simulink model "tuning"  (R2024b)
settings: Solver=FixedStepAuto  StartTime=0.0  StopTime=3  FixedStep=1e-6  RelTol=1e-3
values from neighbouring files (symbols this model uses):
  BW_out = BW_out_DC    [main.m]
  C_filt = parameter.Value(6)    [main.m]
  closedL_P = feedback(openL_P, 1)    [main.m]
  closedL_V = feedback(openL_V, 1)    [main.m]
  DC = 1    [main.m]
  I_charge = C_dc * Vdc_base / t_charge    [main.m]
  inner_loop = collect(-I_V1/V1, "s")    [scam.m]
  ki_outer = ki_outer_DC_pu    [main.m]
  kp_outer = kp_outer_DC_pu    [main.m]
  L_base = Z_base / omega_b    [main.m]
  L_vsc = parameter.Value(5)    [main.m]
  omega_b = 2 * pi * f_base    [main.m]
  P_base = parameter.Value(4)*10^6    [main.m]
  Pm_out = Pm_out_DC    [main.m]
  Power = 0    [main.m]
  R_filt = parameter.Value(8)    [main.m]
  R_vsc = parameter.Value(7)    [main.m]
  t_charge = 0.5    [main.m]
  Ts = parameter.Value(1)*10^-6    [main.m]
  V_base = parameter.Value(3)*10^3    [main.m]
undefined symbols (not defined in the file or in its folder): BW_in, BW_out_DC, BW_out_P, BW_out_V, BW_pll, C_dc, ki_inner_pu, ki_outer_DC_pu, ki_outer_P_pu, ki_outer_V_pu, ki_pll, kp_inner_pu, kp_outer_DC_pu, kp_outer_P_pu, kp_outer_V_pu, kp_pll, L, L_grid, openL_DC, Pm_out_DC, Pm_out_P, Pm_out_V, Pm_pll, R_grid, tau_max, Vdc_base
libraries: slpidlib x5, spsabctodq0Lib x4, spsControlledVoltageSourceLib x3, spsControlledCurrentSourceLib x2, eeGeneralControl x2, spsThreePhaseSeriesRLCBranchLib x2, spsThreePhaseVIMeasurementLib x2, spsGroundLib x1, spsParallelRLCBranchLib x1, spsThreePhaseSourceLib x1, spsVoltageMeasurementLib x1, spsdq0toabcLib x1
settings Model: Creator=osro  LastModifiedBy=nicolae.darii
settings SolverCC: AlgebraicLoopSolver=TrustRegion
settings DebuggingCC: UnconnectedInputMsg=warning  UnconnectedOutputMsg=warning  UnconnectedLineMsg=warning
settings ModelReferenceCC: EnableRefExpFcnMdlSchedulingChecks=on
settings RTWCC: GPUComputeCapability=3.5

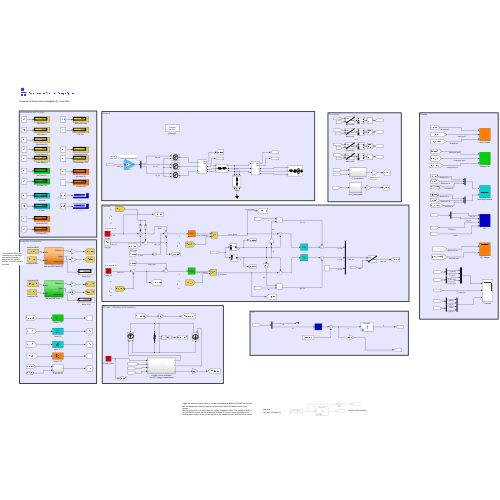
[thumbnail: Simulink's stored preview of the top-level diagram]
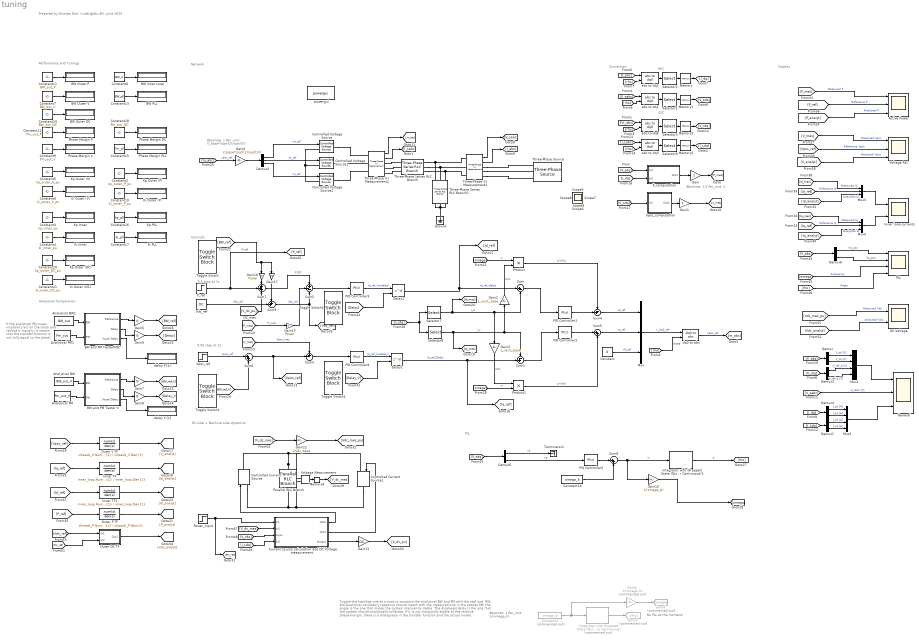
== system tuning ==
  note: PLL
  note: Toggle the switches one at a time to compare the analytical BW and PM with the real one:
      | BW: the analytical oscillatory responce should match with the measured one in the scopes
      | PM: the angle is the one that makes the system margianlly stable. The displayed delay is the one that the system should analytically tollerate. If it is not margianlly stable at the relative phase-margin, there is a divergnece in the transfer function and the actual model.
  note: If the analytical PM cuses instability act on the block and reduce it maualy (it means that the transfer function is not fully equal to the plant)
  note: No PLL at the moment!
  note: 0.05 step at 2s
  note: 0.5 step at 1s
  note: Absolute: 1
      | Per_unit: 1/(omega_b)
  note: Absolute: 1.5
      | Per_unit: 1
  note: Absolute: 1
      | Per_unit: V_base*(sqrt(2)/sqrt(3))
  note: Display
  note: Conversion
  note: Controls
  note: Analytical Comparision
  note: Network
  note: Performance and Tunings
  note: VSC
  note: PoC
  note: Prepared by Nicolae Darii (nidar@dtu.dk), June 2025
  note: DC side + Machine side dynamics
  Active Power : Scope  NumInputPorts=3
  Analytical BW : Constant  Value=BW_out_V
  Analytical BW1 : Constant  Value=BW_out
  Analytical PM : Constant  Value=Pm_out_V
  Analytical PM1 : Constant  Value=Pm_out
  BW Inner Loop : Display
  BW Outer DC : Display
  BW Outer P : Display
  BW Outer V : Display
  BW PLL : Display
  BW and PM Tester V : Subsystem
  BW and PM TesterP/DC : Subsystem
  Constant : Constant  Value=0
  Constant1 : Constant  Commented=on  Value=omega_b
  Constant10 : Constant  Value=ki_outer_P_pu
  Constant11 : Constant  Value=BW_out_P
  Constant12 : Constant  Value=Pm_out_P
  Constant13 : Constant  Value=BW_pll
  Constant14 : Constant  Value=omega_b
  Constant15 : Constant  Value=Pm_pll
  Constant16 : Constant  Value=kp_pll
  Constant17 : Constant  Value=ki_pll
  Constant18 : Constant  Value=Pm_out_DC
  Constant19 : Constant  Value=BW_out_DC
  Constant2 : Constant  Value=kp_outer_P_pu
  Constant20 : Constant  Value=kp_outer_DC_pu
  Constant21 : Constant  Value=ki_outer_DC_pu
  Constant3 : Constant  Value=kp_inner_pu
  Constant4 : Constant  Value=ki_inner_pu
  Constant5 : Constant  Value=kp_outer_V_pu
  Constant6 : Constant  Value=ki_outer_V_pu
  Constant7 : Constant  Value=BW_out_V
  Constant8 : Constant  Value=BW_in
  Constant9 : Constant  Value=Pm_out_V
  Controlled Current Source : spsControlledCurrentSourceLib/Controlled Current Source  Initialize=on  Source_Type=AC  Amplitude=0  Phase=0  Frequency=0  Measurements=None
  Controlled Current Source1 : spsControlledCurrentSourceLib/Controlled Current Source  Initialize=on  Source_Type=AC  Amplitude=0  Phase=0  Frequency=0  Measurements=None
  Controlled Voltage Source : spsControlledVoltageSourceLib/Controlled Voltage Source  Initialize=on  Source_Type=AC  Amplitude=0  Phase=0  Frequency=0  Measurements=None
  Controlled Voltage Source1 : spsControlledVoltageSourceLib/Controlled Voltage Source  Initialize=on  Source_Type=AC  Amplitude=0  Phase=0  Frequency=0  Measurements=None
  Controlled Voltage Source2 : spsControlledVoltageSourceLib/Controlled Voltage Source  Initialize=on  Source_Type=AC  Amplitude=0  Phase=0  Frequency=0  Measurements=None
  Current source calculation and DC Voltage measurement : Subsystem
  DC Voltage : Scope  NumInputPorts=2
  Delay1 : Delay  DelayLengthSource=Input port  DelayLength=floor(tau_max/Ts)  DelayLengthUpperLimit=10000
      settings: InputPortMap=u0,p1
  Delay2 : Delay  DelayLengthSource=Input port  DelayLength=floor(tau_max/Ts)  DelayLengthUpperLimit=10000
      settings: InputPortMap=u0,p1
  Demux{,1,3..6} (6 alike) : Demux  Outputs=2
  Demux2 : Demux  Outputs=3
  Gain : Gain
  Gain1 : Gain
  Gain10 : Gain  Gain=1/(omega_b)
  Gain11 : Gain  Gain=DC
  Gain12 : Gain  Gain=1/Vdc_base
  Gain13 : Gain  Gain=Power
  Gain16 : Gain  Gain=Power
  Gain17 : Gain  Gain=DC
  Gain2 : Gain  Gain=L_vsc/L_base
  Gain3 : Gain  Gain=L_vsc/L_base
  Gain4 : Gain  Commented=on  Gain=1/(omega_b)
  Gain{5,7..9} (4 alike) : Gain  Gain=0
  Gain6 : Gain  Gain=V_base*(sqrt(2)/sqrt(3))
  General : Scope  NumInputPorts=3
  Goto3 : Goto  Commented=on  GotoTag=rho
  Goto4 : Goto  Commented=on  GotoTag=omega
  Ground : spsGroundLib/Ground  LConnTagsString=a
  Inner TF : TransferFcn  Numerator=inner_loop.Num{1}  Denominator=inner_loop.Den{1}
  Inner TF1 : TransferFcn  Numerator=inner_loop.Num{1}  Denominator=inner_loop.Den{1}
  Inner loop currents : Scope  NumInputPorts=2
  Integrator with Wrapped State (Discrete or Continuous) : eeGeneralControl/Integrator with Wrapped State (Discrete or Continuous)  Commented=on  LabelModeActiveChoice=Discrete  WrappedStateUpperValue=2*pi  WrappedStateLowerValue=0  x0=0  Ts=-1
  Integrator with Wrapped State (Discrete or Continuous)1 : eeGeneralControl/Integrator with Wrapped State (Discrete or Continuous)  LabelModeActiveChoice=Discrete  WrappedStateUpperValue=2*pi  WrappedStateLowerValue=0  x0=0  Ts=-1
  Ki Inner : Display
  Ki Outer (DC) : Display
  Ki Outer (P) : Display
  Ki Outer (V) : Display
  Ki PLL : Display
  Kp Inner : Display
  Kp Outer (DC) : Display
  Kp Outer (P) : Display
  Kp Outer (V) : Display
  Kp PLL : Display
  Memory{,1..3} (4 alike) : Memory  InitialCondition=[0 0]  InheritSampleTime=on  LinearizeMemory=on  LinearizeAsDelay=on
  Memory4 : Memory
  Mux : Mux  Inputs=3
  Mux1 : Mux
  Mux2 : Mux
  Mux3 : Mux  Inputs=3
  Mux4 : Mux  Inputs=3
  Outer DC TF : Subsystem
  Outer P TF : TransferFcn  Numerator=closedL_P.Num{1}  Denominator=closedL_P.Den{1}
  Outer V TF : TransferFcn  Numerator=closedL_V.Num{1}  Denominator=closedL_V.Den{1}
  PID Controller1 : slpidlib/PID Controller  Controller=PI  Form=Parallel  TimeDomain=Discrete-time  UseExternalTs=off  SampleTime=Ts  IntegratorMethod=Forward Euler  FilterMethod=Forward Euler  ControllerParametersSource=internal  P=kp_inner_pu  I=ki_inner_pu  UseKiTs=off  D=0  UseExternalDerivativeSource=off  N=100  UseFilter=on  TunerSelectOption=Transfer Function Based (PID Tuner App)  InitialConditionSource=internal  InitialConditionForIntegrator=0  InitialConditionForFilter=0  DifferentiatorICPrevScaledInput=0  ExternalReset=none  TrackingMode=off  Kt=1  LimitOutput=off  SatLimitsSource=internal  UpperSaturationLimit=inf  LowerSaturationLimit=-inf  LinearizeAsGain=on  AntiWindupMode=none  Kb=1  LimitIntegrator=off  UpperIntegratorSaturationLimit=inf  LowerIntegratorSaturationLimit=-inf  POutMin=[]  POutMax=[]  IOutMin=[]  IOutMax=[]  DOutMin=[]  DOutMax=[]  NOutMin=[]  NOutMax=[]  SumOutMin=[]  SumOutMax=[]  SaturationOutMin=[]  SaturationOutMax=[]  PParamMin=[]  PParamMax=[]  IParamMin=[]  IParamMax=[]  DParamMin=[]  DParamMax=[]  NParamMin=[]  NParamMax=[]  KbParamMin=[]  KbParamMax=[]  KtParamMin=[]  KtParamMax=[]  KbOutMin=[]  KbOutMax=[]  KtOutMin=[]  KtOutMax=[]  IntegratorOutMin=[]  IntegratorOutMax=[]  FilterOutMin=[]  FilterOutMax=[]  SumI1OutMin=[]  SumI1OutMax=[]  SumI2OutMin=[]  SumI2OutMax=[]  SumI3OutMin=[]  SumI3OutMax=[]  SumI4OutMin=[]  SumI4OutMax=[]  SumDOutMin=[]  SumDOutMax=[]  DifferentiatorOutMin=[]  DifferentiatorOutMax=[]  FilterDiffOutCoefMin=[]  FilterDiffOutCoefMax=[]  ReciprocalOutMin=[]  ReciprocalOutMax=[]  SumDenOutMin=[]  SumDenOutMax=[]  SumNumOutMin=[]  SumNumOutMax=[]  DivideOutMin=[]  DivideOutMax=[]  UdiffTsProdOutMin=[]  UdiffTsProdOutMax=[]  NTsProdOutMin=[]  NTsProdOutMax=[]  UintegralTsProdOutMin=[]  UintegralTsProdOutMax=[]  UngainTsProdOutMin=[]  UngainTsProdOutMax=[]  ClampingZeroOutDataTypeStr=Inherit: Inherit via back propagation  ClampingZeroOutMin=[]  ClampingZeroOutMax=[]  FilterDenConstantOutDataTypeStr=Inherit: Inherit via back propagation  FilterDenConstantOutMin=[]  FilterDenConstantOutMax=[]  PCopyOutDataTypeStr=Inherit: Inherit via back propagation  PCopyOutMin=[]  PCopyOutMax=[]  NCopyOutDataTypeStr=Inherit: Inherit via back propagation  NCopyOutMin=[]  NCopyOutMax=[]  IntegratorContinuousStateAttributes=''  IntegratorStateMustResolveToSignalObject=off  IntegratorRTWStateStorageClass=Auto  FilterContinuousStateAttributes=''  FilterStateMustResolveToSignalObject=off  FilterRTWStateStorageClass=Auto  ParallelPVariant=InternalParameters  IdealPVariant=Disabled  IVariant=InternalParameters  DVariant=Disabled  IntegratorVariant=Discrete  SatVariant=Disabled  AWVariant=Passthrough  PCopyVariant=Disabled  TRVariant=Disabled  FdbkBlocksVariant=Forward  IdealPFdbkVariant=Disabled  SatFdbkVariant=Disabled  DerivativeFilterVariant=Disabled  NVariant=Disabled  NCopyVariant=Disabled_SignalSpec  FilterICVariant=Disabled  IntegratorICVariant=InternalICs  ExternalResetVariant=Disabled  TRSumVariant=Passthrough  SumFdbkVariant=Disabled  SumVariant=Sum_PI  TsampFilterVariant=InternalTs  TsampNgainVariant=Passthrough  TsampIntegralVariant=Disabled_SignalSpec  ExternalSaturationOutDataTypeStr=Inherit: Same as second input  DerivativeSourceVariant=Disabled  PreIntVariant=InternalPreInt
  PID Controller2 : slpidlib/PID Controller  Controller=PI  Form=Parallel  TimeDomain=Discrete-time  UseExternalTs=off  SampleTime=Ts  IntegratorMethod=Forward Euler  FilterMethod=Forward Euler  ControllerParametersSource=internal  P=kp_inner_pu  I=ki_inner_pu  UseKiTs=off  D=0  UseExternalDerivativeSource=off  N=100  UseFilter=on  TunerSelectOption=Transfer Function Based (PID Tuner App)  InitialConditionSource=internal  InitialConditionForIntegrator=0  InitialConditionForFilter=0  DifferentiatorICPrevScaledInput=0  ExternalReset=none  TrackingMode=off  Kt=1  LimitOutput=off  SatLimitsSource=internal  UpperSaturationLimit=inf  LowerSaturationLimit=-inf  LinearizeAsGain=on  AntiWindupMode=none  Kb=1  LimitIntegrator=off  UpperIntegratorSaturationLimit=inf  LowerIntegratorSaturationLimit=-inf  POutMin=[]  POutMax=[]  IOutMin=[]  IOutMax=[]  DOutMin=[]  DOutMax=[]  NOutMin=[]  NOutMax=[]  SumOutMin=[]  SumOutMax=[]  SaturationOutMin=[]  SaturationOutMax=[]  PParamMin=[]  PParamMax=[]  IParamMin=[]  IParamMax=[]  DParamMin=[]  DParamMax=[]  NParamMin=[]  NParamMax=[]  KbParamMin=[]  KbParamMax=[]  KtParamMin=[]  KtParamMax=[]  KbOutMin=[]  KbOutMax=[]  KtOutMin=[]  KtOutMax=[]  IntegratorOutMin=[]  IntegratorOutMax=[]  FilterOutMin=[]  FilterOutMax=[]  SumI1OutMin=[]  SumI1OutMax=[]  SumI2OutMin=[]  SumI2OutMax=[]  SumI3OutMin=[]  SumI3OutMax=[]  SumI4OutMin=[]  SumI4OutMax=[]  SumDOutMin=[]  SumDOutMax=[]  DifferentiatorOutMin=[]  DifferentiatorOutMax=[]  FilterDiffOutCoefMin=[]  FilterDiffOutCoefMax=[]  ReciprocalOutMin=[]  ReciprocalOutMax=[]  SumDenOutMin=[]  SumDenOutMax=[]  SumNumOutMin=[]  SumNumOutMax=[]  DivideOutMin=[]  DivideOutMax=[]  UdiffTsProdOutMin=[]  UdiffTsProdOutMax=[]  NTsProdOutMin=[]  NTsProdOutMax=[]  UintegralTsProdOutMin=[]  UintegralTsProdOutMax=[]  UngainTsProdOutMin=[]  UngainTsProdOutMax=[]  ClampingZeroOutDataTypeStr=Inherit: Inherit via back propagation  ClampingZeroOutMin=[]  ClampingZeroOutMax=[]  FilterDenConstantOutDataTypeStr=Inherit: Inherit via back propagation  FilterDenConstantOutMin=[]  FilterDenConstantOutMax=[]  PCopyOutDataTypeStr=Inherit: Inherit via back propagation  PCopyOutMin=[]  PCopyOutMax=[]  NCopyOutDataTypeStr=Inherit: Inherit via back propagation  NCopyOutMin=[]  NCopyOutMax=[]  IntegratorContinuousStateAttributes=''  IntegratorStateMustResolveToSignalObject=off  IntegratorRTWStateStorageClass=Auto  FilterContinuousStateAttributes=''  FilterStateMustResolveToSignalObject=off  FilterRTWStateStorageClass=Auto  ParallelPVariant=InternalParameters  IdealPVariant=Disabled  IVariant=InternalParameters  DVariant=Disabled  IntegratorVariant=Discrete  SatVariant=Disabled  AWVariant=Passthrough  PCopyVariant=Disabled  TRVariant=Disabled  FdbkBlocksVariant=Forward  IdealPFdbkVariant=Disabled  SatFdbkVariant=Disabled  DerivativeFilterVariant=Disabled  NVariant=Disabled  NCopyVariant=Disabled_SignalSpec  FilterICVariant=Disabled  IntegratorICVariant=InternalICs  ExternalResetVariant=Disabled  TRSumVariant=Passthrough  SumFdbkVariant=Disabled  SumVariant=Sum_PI  TsampFilterVariant=InternalTs  TsampNgainVariant=Passthrough  TsampIntegralVariant=Disabled_SignalSpec  ExternalSaturationOutDataTypeStr=Inherit: Same as second input  DerivativeSourceVariant=Disabled  PreIntVariant=InternalPreInt
  PID Controller3 : slpidlib/PID Controller  Controller=PI  Form=Parallel  TimeDomain=Discrete-time  UseExternalTs=off  SampleTime=Ts  IntegratorMethod=Forward Euler  FilterMethod=Forward Euler  ControllerParametersSource=internal  P=kp_outer  I=ki_outer  UseKiTs=off  D=0  UseExternalDerivativeSource=off  N=100  UseFilter=on  TunerSelectOption=Transfer Function Based (PID Tuner App)  InitialConditionSource=internal  InitialConditionForIntegrator=0  InitialConditionForFilter=0  DifferentiatorICPrevScaledInput=0  ExternalReset=none  TrackingMode=off  Kt=1  LimitOutput=off  SatLimitsSource=internal  UpperSaturationLimit=inf  LowerSaturationLimit=-inf  LinearizeAsGain=on  AntiWindupMode=none  Kb=1  LimitIntegrator=off  UpperIntegratorSaturationLimit=inf  LowerIntegratorSaturationLimit=-inf  POutMin=[]  POutMax=[]  IOutMin=[]  IOutMax=[]  DOutMin=[]  DOutMax=[]  NOutMin=[]  NOutMax=[]  SumOutMin=[]  SumOutMax=[]  SaturationOutMin=[]  SaturationOutMax=[]  PParamMin=[]  PParamMax=[]  IParamMin=[]  IParamMax=[]  DParamMin=[]  DParamMax=[]  NParamMin=[]  NParamMax=[]  KbParamMin=[]  KbParamMax=[]  KtParamMin=[]  KtParamMax=[]  KbOutMin=[]  KbOutMax=[]  KtOutMin=[]  KtOutMax=[]  IntegratorOutMin=[]  IntegratorOutMax=[]  FilterOutMin=[]  FilterOutMax=[]  SumI1OutMin=[]  SumI1OutMax=[]  SumI2OutMin=[]  SumI2OutMax=[]  SumI3OutMin=[]  SumI3OutMax=[]  SumI4OutMin=[]  SumI4OutMax=[]  SumDOutMin=[]  SumDOutMax=[]  DifferentiatorOutMin=[]  DifferentiatorOutMax=[]  FilterDiffOutCoefMin=[]  FilterDiffOutCoefMax=[]  ReciprocalOutMin=[]  ReciprocalOutMax=[]  SumDenOutMin=[]  SumDenOutMax=[]  SumNumOutMin=[]  SumNumOutMax=[]  DivideOutMin=[]  DivideOutMax=[]  UdiffTsProdOutMin=[]  UdiffTsProdOutMax=[]  NTsProdOutMin=[]  NTsProdOutMax=[]  UintegralTsProdOutMin=[]  UintegralTsProdOutMax=[]  UngainTsProdOutMin=[]  UngainTsProdOutMax=[]  ClampingZeroOutDataTypeStr=Inherit: Inherit via back propagation  ClampingZeroOutMin=[]  ClampingZeroOutMax=[]  FilterDenConstantOutDataTypeStr=Inherit: Inherit via back propagation  FilterDenConstantOutMin=[]  FilterDenConstantOutMax=[]  PCopyOutDataTypeStr=Inherit: Inherit via back propagation  PCopyOutMin=[]  PCopyOutMax=[]  NCopyOutDataTypeStr=Inherit: Inherit via back propagation  NCopyOutMin=[]  NCopyOutMax=[]  IntegratorContinuousStateAttributes=''  IntegratorStateMustResolveToSignalObject=off  IntegratorRTWStateStorageClass=Auto  FilterContinuousStateAttributes=''  FilterStateMustResolveToSignalObject=off  FilterRTWStateStorageClass=Auto  ParallelPVariant=InternalParameters  IdealPVariant=Disabled  IVariant=InternalParameters  DVariant=Disabled  IntegratorVariant=Discrete  SatVariant=Disabled  AWVariant=Passthrough  PCopyVariant=Disabled  TRVariant=Disabled  FdbkBlocksVariant=Forward  IdealPFdbkVariant=Disabled  SatFdbkVariant=Disabled  DerivativeFilterVariant=Disabled  NVariant=Disabled  NCopyVariant=Disabled_SignalSpec  FilterICVariant=Disabled  IntegratorICVariant=InternalICs  ExternalResetVariant=Disabled  TRSumVariant=Passthrough  SumFdbkVariant=Disabled  SumVariant=Sum_PI  TsampFilterVariant=InternalTs  TsampNgainVariant=Passthrough  TsampIntegralVariant=Disabled_SignalSpec  ExternalSaturationOutDataTypeStr=Inherit: Same as second input  DerivativeSourceVariant=Disabled  PreIntVariant=InternalPreInt
  PID Controller4 : slpidlib/PID Controller  Controller=PI  Form=Parallel  TimeDomain=Discrete-time  UseExternalTs=off  SampleTime=Ts  IntegratorMethod=Forward Euler  FilterMethod=Forward Euler  ControllerParametersSource=internal  P=abs(kp_outer_V_pu)  I=abs(ki_outer_V_pu)  UseKiTs=off  D=0  UseExternalDerivativeSource=off  N=100  UseFilter=on  TunerSelectOption=Transfer Function Based (PID Tuner App)  InitialConditionSource=internal  InitialConditionForIntegrator=0  InitialConditionForFilter=0  DifferentiatorICPrevScaledInput=0  ExternalReset=none  TrackingMode=off  Kt=1  LimitOutput=off  SatLimitsSource=internal  UpperSaturationLimit=inf  LowerSaturationLimit=-inf  LinearizeAsGain=on  AntiWindupMode=none  Kb=1  LimitIntegrator=off  UpperIntegratorSaturationLimit=inf  LowerIntegratorSaturationLimit=-inf  POutMin=[]  POutMax=[]  IOutMin=[]  IOutMax=[]  DOutMin=[]  DOutMax=[]  NOutMin=[]  NOutMax=[]  SumOutMin=[]  SumOutMax=[]  SaturationOutMin=[]  SaturationOutMax=[]  PParamMin=[]  PParamMax=[]  IParamMin=[]  IParamMax=[]  DParamMin=[]  DParamMax=[]  NParamMin=[]  NParamMax=[]  KbParamMin=[]  KbParamMax=[]  KtParamMin=[]  KtParamMax=[]  KbOutMin=[]  KbOutMax=[]  KtOutMin=[]  KtOutMax=[]  IntegratorOutMin=[]  IntegratorOutMax=[]  FilterOutMin=[]  FilterOutMax=[]  SumI1OutMin=[]  SumI1OutMax=[]  SumI2OutMin=[]  SumI2OutMax=[]  SumI3OutMin=[]  SumI3OutMax=[]  SumI4OutMin=[]  SumI4OutMax=[]  SumDOutMin=[]  SumDOutMax=[]  DifferentiatorOutMin=[]  DifferentiatorOutMax=[]  FilterDiffOutCoefMin=[]  FilterDiffOutCoefMax=[]  ReciprocalOutMin=[]  ReciprocalOutMax=[]  SumDenOutMin=[]  SumDenOutMax=[]  SumNumOutMin=[]  SumNumOutMax=[]  DivideOutMin=[]  DivideOutMax=[]  UdiffTsProdOutMin=[]  UdiffTsProdOutMax=[]  NTsProdOutMin=[]  NTsProdOutMax=[]  UintegralTsProdOutMin=[]  UintegralTsProdOutMax=[]  UngainTsProdOutMin=[]  UngainTsProdOutMax=[]  ClampingZeroOutDataTypeStr=Inherit: Inherit via back propagation  ClampingZeroOutMin=[]  ClampingZeroOutMax=[]  FilterDenConstantOutDataTypeStr=Inherit: Inherit via back propagation  FilterDenConstantOutMin=[]  FilterDenConstantOutMax=[]  PCopyOutDataTypeStr=Inherit: Inherit via back propagation  PCopyOutMin=[]  PCopyOutMax=[]  NCopyOutDataTypeStr=Inherit: Inherit via back propagation  NCopyOutMin=[]  NCopyOutMax=[]  IntegratorContinuousStateAttributes=''  IntegratorStateMustResolveToSignalObject=off  IntegratorRTWStateStorageClass=Auto  FilterContinuousStateAttributes=''  FilterStateMustResolveToSignalObject=off  FilterRTWStateStorageClass=Auto  ParallelPVariant=InternalParameters  IdealPVariant=Disabled  IVariant=InternalParameters  DVariant=Disabled  IntegratorVariant=Discrete  SatVariant=Disabled  AWVariant=Passthrough  PCopyVariant=Disabled  TRVariant=Disabled  FdbkBlocksVariant=Forward  IdealPFdbkVariant=Disabled  SatFdbkVariant=Disabled  DerivativeFilterVariant=Disabled  NVariant=Disabled  NCopyVariant=Disabled_SignalSpec  FilterICVariant=Disabled  IntegratorICVariant=InternalICs  ExternalResetVariant=Disabled  TRSumVariant=Passthrough  SumFdbkVariant=Disabled  SumVariant=Sum_PI  TsampFilterVariant=InternalTs  TsampNgainVariant=Passthrough  TsampIntegralVariant=Disabled_SignalSpec  ExternalSaturationOutDataTypeStr=Inherit: Same as second input  DerivativeSourceVariant=Disabled  PreIntVariant=InternalPreInt
  PID Controller5 : slpidlib/PID Controller  Controller=PI  Form=Parallel  TimeDomain=Discrete-time  UseExternalTs=off  SampleTime=Ts  IntegratorMethod=Forward Euler  FilterMethod=Forward Euler  ControllerParametersSource=internal  P=kp_pll  I=ki_pll  UseKiTs=off  D=0  UseExternalDerivativeSource=off  N=100  UseFilter=on  TunerSelectOption=Transfer Function Based (PID Tuner App)  InitialConditionSource=internal  InitialConditionForIntegrator=0  InitialConditionForFilter=0  DifferentiatorICPrevScaledInput=0  ExternalReset=none  TrackingMode=off  Kt=1  LimitOutput=off  SatLimitsSource=internal  UpperSaturationLimit=inf  LowerSaturationLimit=-inf  LinearizeAsGain=on  AntiWindupMode=none  Kb=1  LimitIntegrator=off  UpperIntegratorSaturationLimit=inf  LowerIntegratorSaturationLimit=-inf  POutMin=[]  POutMax=[]  IOutMin=[]  IOutMax=[]  DOutMin=[]  DOutMax=[]  NOutMin=[]  NOutMax=[]  SumOutMin=[]  SumOutMax=[]  SaturationOutMin=[]  SaturationOutMax=[]  PParamMin=[]  PParamMax=[]  IParamMin=[]  IParamMax=[]  DParamMin=[]  DParamMax=[]  NParamMin=[]  NParamMax=[]  KbParamMin=[]  KbParamMax=[]  KtParamMin=[]  KtParamMax=[]  KbOutMin=[]  KbOutMax=[]  KtOutMin=[]  KtOutMax=[]  IntegratorOutMin=[]  IntegratorOutMax=[]  FilterOutMin=[]  FilterOutMax=[]  SumI1OutMin=[]  SumI1OutMax=[]  SumI2OutMin=[]  SumI2OutMax=[]  SumI3OutMin=[]  SumI3OutMax=[]  SumI4OutMin=[]  SumI4OutMax=[]  SumDOutMin=[]  SumDOutMax=[]  DifferentiatorOutMin=[]  DifferentiatorOutMax=[]  FilterDiffOutCoefMin=[]  FilterDiffOutCoefMax=[]  ReciprocalOutMin=[]  ReciprocalOutMax=[]  SumDenOutMin=[]  SumDenOutMax=[]  SumNumOutMin=[]  SumNumOutMax=[]  DivideOutMin=[]  DivideOutMax=[]  UdiffTsProdOutMin=[]  UdiffTsProdOutMax=[]  NTsProdOutMin=[]  NTsProdOutMax=[]  UintegralTsProdOutMin=[]  UintegralTsProdOutMax=[]  UngainTsProdOutMin=[]  UngainTsProdOutMax=[]  ClampingZeroOutDataTypeStr=Inherit: Inherit via back propagation  ClampingZeroOutMin=[]  ClampingZeroOutMax=[]  FilterDenConstantOutDataTypeStr=Inherit: Inherit via back propagation  FilterDenConstantOutMin=[]  FilterDenConstantOutMax=[]  PCopyOutDataTypeStr=Inherit: Inherit via back propagation  PCopyOutMin=[]  PCopyOutMax=[]  NCopyOutDataTypeStr=Inherit: Inherit via back propagation  NCopyOutMin=[]  NCopyOutMax=[]  IntegratorContinuousStateAttributes=''  IntegratorStateMustResolveToSignalObject=off  IntegratorRTWStateStorageClass=Auto  FilterContinuousStateAttributes=''  FilterStateMustResolveToSignalObject=off  FilterRTWStateStorageClass=Auto  ParallelPVariant=InternalParameters  IdealPVariant=Disabled  IVariant=InternalParameters  DVariant=Disabled  IntegratorVariant=Discrete  SatVariant=Disabled  AWVariant=Passthrough  PCopyVariant=Disabled  TRVariant=Disabled  FdbkBlocksVariant=Forward  IdealPFdbkVariant=Disabled  SatFdbkVariant=Disabled  DerivativeFilterVariant=Disabled  NVariant=Disabled  NCopyVariant=Disabled_SignalSpec  FilterICVariant=Disabled  IntegratorICVariant=InternalICs  ExternalResetVariant=Disabled  TRSumVariant=Passthrough  SumFdbkVariant=Disabled  SumVariant=Sum_PI  TsampFilterVariant=InternalTs  TsampNgainVariant=Passthrough  TsampIntegralVariant=Disabled_SignalSpec  ExternalSaturationOutDataTypeStr=Inherit: Same as second input  DerivativeSourceVariant=Disabled  PreIntVariant=InternalPreInt
  PLL : Scope  NumInputPorts=4
  P_computation : Subsystem
  P_ref : Step  After=0.5*Power  SampleTime=0
  Parallel RLC Branch : spsParallelRLCBranchLib/Parallel RLC Branch  LConnTagsString=a  RConnTagsString=__new0  BranchType=C  Resistance=1  Inductance=1e-3  SetiL0=off  InitialCurrent=0  Capacitance=C_dc  Setx0=on  InitialVoltage=0  Measurements=None
  Phase Margin DC : Display
  Phase Margin P : Display
  Phase Margin PLL : Display
  Phase Margin V : Display
  Power_Input : Step  After=0.5*DC  SampleTime=0
  Product : Product
  Product1 : Product
  Selector{1..3,9} (4 alike) : Selector  InputPortWidth=3  IndexOptions=Index vector (dialog)  Indices=[1 2]  OutputSizes=1
  Selector7 : Selector  InputPortWidth=2  IndexOptions=Index vector (dialog)  Indices=[1]  OutputSizes=1
  Selector8 : Selector  InputPortWidth=2  IndexOptions=Index vector (dialog)  Indices=[2]  OutputSizes=1
  Sum : Sum  Inputs=|+-
  Sum1 : Sum  Inputs=-+|
  Sum2 : Sum  Inputs=+--
  Sum3 : Sum  Inputs=+-|
  Sum4 : Sum  Inputs=-+|
  Sum5 : Sum  Inputs=|++
  Sum6 : Sum  Inputs=|++
  Sum7 : Sum  Inputs=+++
  Sum8 : Sum  Inputs=|++
  Sum9 : Sum  Inputs=++|
  Terminator1 : Terminator
  Three-Phase Series RLC Branch : spsThreePhaseSeriesRLCBranchLib/Three-Phase Series RLC Branch  LConnTagsString=A|B|C  RConnTagsString=A|B|C  BranchType=RL  Resistance=R_vsc  Inductance=L_vsc  Capacitance=1e-6  Measurements=None
  Three-Phase Series RLC Branch1 : spsThreePhaseSeriesRLCBranchLib/Three-Phase Series RLC Branch  LConnTagsString=A|B|C  RConnTagsString=A|B|C  BranchType=RC  Resistance=R_filt  Inductance=L  Capacitance=C_filt  Measurements=None
  Three-Phase V-I Measurement1 : spsThreePhaseVIMeasurementLib/Three-Phase V-I Measurement  VoltageMeasurement=phase-to-ground  SetLabelV=off  LabelV=Vabc  Vpu=on  VpuLL=off  CurrentMeasurement=yes  SetLabelI=off  LabelI=Iabc  Ipu=on  Pbase=P_base  Vbase=V_base  OutputType=Complex  PhasorSimulation=off  PSBequivalent=0
  Three-Phase V-I Measurement2 : spsThreePhaseVIMeasurementLib/Three-Phase V-I Measurement  VoltageMeasurement=phase-to-ground  SetLabelV=off  LabelV=Vabc  Vpu=on  VpuLL=off  CurrentMeasurement=yes  SetLabelI=off  LabelI=Iabc  Ipu=on  Pbase=P_base  Vbase=V_base  OutputType=Complex  PhasorSimulation=off  PSBequivalent=0
  Three-Phase Source : spsThreePhaseSourceLib/Three-Phase Source  InternalConnection=Yg  VoltagePhases=off  Voltage=V_base  PhaseAngle=0  Voltage_phases=[25e3 25e3 25e3]/sqrt(3)  PhaseAngles_phases=[0 -120 +120]  Frequency=50  NonIdealSource=on  SpecifyImpedance=off  Resistance=R_grid  Inductance=L_grid  ShortCircuitLevel=100e6  BaseVoltage=V_base  XRratio=7  BusType=swing  Pref=10e3  Qref=0  Prefabc=[10e3, 10e3, 10e3]  Qrefabc=[0, 0, 0]  Qmin=-inf  Qmax=inf
  Toggle Switch{,1..2,4} (4 alike) : ToggleSwitchBlock  LabelPosition=Hide
      settings: Values={{'Off', 'On'}, [0 1]}
  Vdc_ref : Constant  Value=DC
  Voltage Measurement : spsVoltageMeasurementLib/Voltage Measurement  PhasorSimulation=off  OutputType=Complex  PSBequivalent=0
  Voltage PoC : Scope  NumInputPorts=3
  Vpoc_computation : Subsystem
  Vpoc_ref : Step  Time=2  Before=1  After=1.05  SampleTime=0
  abc to dq{1..4} (4 alike) : spsabctodq0Lib/abc to dq0  Alignment=90 degrees behind phase A axis
  delay P [s] : Display
  delay V [s] : Display
  dq0 to abc : spsdq0toabcLib/dq0 to abc  Alignment=90 degrees behind phase A axis
  powergui : sps_lib/powergui  Priority=1  SimulationMode=Discrete  SampleTime=Ts  frequency=60  Iterations=50  frequencyindice=0  Pbase=100e6  ErrMax=1e-4  UnitsV=kV  UnitsW=MW  buscounter=0  FunctionMessages=off  echomessages=off  EnableUseOfTLC=off  CurrentSourceSwitches=off  DisableSnubberDevices=off  DisableRonSwitches=off  DisableVfSwitches=off  DisplayEquations=off  AutomaticDiscreteSolvers=off  SolverType=Tustin/Backward Euler (TBE)  Interpol=off  ExternalGateDelay=off  methode=off  Ts=100  x0status=zero  SPID=on  SwTol=0  HookPort=off  NonlinearTolerance=1e-4  nMaxIteration=100  ContinueOnMaxIteration=off  RestoreLinks=warning  ResistiveCurrentMeasurement=off  Frange=[0:2:500]  Ylog=off  Xlog=on  ShowGrid=off  save=off  variable=ZData  structure=0  ZoomFFT=off  StartTime=0.0  cycles=1  DisplayStyle=1  fundamental=60  FreqAxis=off  MaxFrequency=1000  frequencyindicesteady=1  RmsSteady=1  display=off
  Scope{2,5..9} (6 alike) : Scope
  wires:
  Selector1/1 -> Memory1/1
  abc to dq1/1 -> Selector1/1
  Constant1/1 -> Integrator with Wrapped State (Discrete or Continuous)/1, Gain4/1
  [rho] -> dq0 to abc/2  "theta"
  [V_sabc] -> abc to dq1/1
  [rho] -> abc to dq1/2
  [rho] -> abc to dq2/2
  Selector2/1 -> Memory/1
  [I_abc] -> abc to dq2/1
  abc to dq2/1 -> Selector2/1
  Constant/1 -> Mux/3  "v0_ref"
  [V_sabc] -> General/2  "V_sabc [V]"
  Three-Phase V-I Measurement1/2 -> [I_Labc]
  Memory/1 -> [I_dq]
  Memory1/1 -> [V_sdq]
  Integrator with Wrapped State (Discrete or Continuous)/1 -> Goto3/1
  Mux2/1 -> General/3
  Three-Phase V-I Measurement2/1 -> [V_sabc]
  Three-Phase V-I Measurement2/2 -> [I_abc]
  Memory2/1 -> [I_Ldq]
  abc to dq3/1 -> Selector9/1
  [I_Labc] -> abc to dq3/1
  Selector9/1 -> Memory2/1
  [rho] -> abc to dq3/2
  Demux/1 -> Mux1/1  "V_sd [V]"
  Demux/2 -> Mux1/2  "V_sq [V]"
  [V_sdq] -> Demux/1
  Mux1/1 -> General/1
  [I_Ldq] -> Demux1/1
  [V_sdq] -> P_computation/1(In1)
  [I_dq] -> P_computation/2(In2)
  P_computation/1(Out1) -> Gain/1
  [V_sdq] -> Vpoc_computation/1(In1)
  Vpoc_computation/1(Out1) -> Gain1/1
  Gain6/1 -> Demux2/1
  Demux2/1 -> Controlled Voltage Source/1  "va_ref"
  Demux2/2 -> Controlled Voltage Source1/1  "vb_ref"
  Demux2/3 -> Controlled Voltage Source2/1  "vc_ref"
  Three-Phase V-I Measurement1/1 -> [Vr_abc]
  [m_abc] -> Gain6/1  "vabc_ref"
  Selector7/1 -> [Id_mes], Sum/2, Gain3/1  "I_d"
  [I_Ldq] -> Selector8/1, Selector7/1
  Selector8/1 -> [Iq_mes], Sum1/1, Gain2/1  "I_q"
  Sum/1 -> PID Controller1/1
  Sum1/1 -> PID Controller2/1
  [rho] -> abc to dq4/2
  Selector3/1 -> Memory3/1
  Memory3/1 -> [V_rdq]
  abc to dq4/1 -> Selector3/1
  [Vr_abc] -> abc to dq4/1
  [V_rdq] -> Demux3/1
  Demux3/1 -> Mux1/3  "V_ref_d [V]"
  Demux3/2 -> Mux1/4  "V_ref_q [V]"
  [I_dq] -> Demux4/1
  Demux1/1 -> Mux2/3  "I_Ld [A]"
  Demux1/2 -> Mux2/4  "I_Lq [A]"
  Demux4/1 -> Mux2/1  "I_sd [A]"
  Demux4/2 -> Mux2/2  "I_sq [A]"
  Sum2/1 -> PID Controller3/1
  Sum3/1 -> PID Controller4/1
  [V_mes] -> Sum3/1  "Vpoc_mes"
  Vpoc_ref/1 -> Sum6/1  "Vpoc_ref"
  dq0 to abc/1 -> [m_abc]  "vabc_ref"
  Constant3/1 -> Kp Inner/1
  Constant4/1 -> Ki Inner/1
  Constant5/1 -> Kp Outer (V)/1
  Constant6/1 -> Ki Outer (V)/1
  Gain/1 -> [P_mes]
  Gain1/1 -> [V_mes]
  PID Controller4/1 -> Delay1/1  "Iq_ref_(nodelay)"
  [omega] -> Product/1  "w"
  Gain2/1 -> Product/2  "Iq*L"
  [omega] -> Product1/2  "w"
  Gain3/1 -> Product1/1  "Id*L"
  PID Controller1/1 -> Sum4/2
  Sum4/1 -> Mux/1  "vd_ref"
  Product/1 -> Sum4/1  "w*L*Iq"
  PID Controller2/1 -> Sum5/1
  Sum5/1 -> Mux/2  "vq_ref"
  Product1/1 -> Sum5/2  "w*L*Id"
  Sum6/1 -> [Vpoc_ref], Sum3/2
  [V_mes] -> Voltage PoC/1  "Measured Vpoc"
  [Vpoc_ref] -> Voltage PoC/2  "Reference Vpoc"
  [Delay_V] -> Delay1/2
  Gain8/1 -> [Delay_V]
  Constant7/1 -> BW Outer V/1
  Constant8/1 -> BW Inner Loop/1
  Constant9/1 -> Phase Margin V/1
  Analytical BW/1 -> BW and PM Tester V/1(BW)
  Analytical PM/1 -> BW and PM Tester V/2(PM)
  BW and PM Tester V/1(Reference) -> Gain7/1
  BW and PM Tester V/2(Delay) -> Gain8/1
  Gain7/1 -> [BW_ref_V]
  [BW_ref_V] -> Sum6/2
  [V_analyt] -> Voltage PoC/3  "Analytical Vpoc"
  Delay1/1 -> [Iq_ref], Sum1/2  "Iq_ref_Delay"
  Gain4/1 -> Goto4/1
  [Vpoc_ref] -> Outer V TF/1
  Outer V TF/1 -> [V_analyt]
  [Iq_ref] -> Inner TF/1
  Inner TF/1 -> [Iq_analyt]
  Delay2/1 -> [Id_ref], Sum/1  "Id_ref_Delay"
  [P_ref] -> Outer P TF/1
  Outer P TF/1 -> [P_analyt]
  [P_mes] -> Active Power/1  "Measured P"
  [P_analyt] -> Active Power/3  "Analytical P"
  [P_ref] -> Active Power/2  "Reference P"
  [Id_ref] -> Inner TF1/1
  Inner TF1/1 -> [Id_analyt]
  [Id_mes] -> Mux3/1  "Measured Id"
  [Id_ref] -> Mux3/2  "Reference Id"
  [Id_analyt] -> Mux3/3  "Anaytical Id"
  Mux3/1 -> Inner loop currents/1
  [Iq_ref] -> Mux4/2  "Reference Iq"
  [Iq_mes] -> Mux4/1  "Measured Iq"
  [Iq_analyt] -> Mux4/3  "Analytical Iq"
  Mux4/1 -> Inner loop currents/2
  Constant2/1 -> Kp Outer (P)/1
  Constant10/1 -> Ki Outer (P)/1
  Constant11/1 -> BW Outer P/1
  Constant12/1 -> Phase Margin P/1
  Analytical BW1/1 -> BW and PM TesterP/DC/1(BW)
  BW and PM TesterP/DC/2(Delay) -> Gain9/1
  Gain5/1 -> [BW_ref]
  BW and PM TesterP/DC/1(Reference) -> Gain5/1
  Analytical PM1/1 -> BW and PM TesterP/DC/2(PM)
  Gain9/1 -> [Delay]
  [BW_ref] -> Gain16/1, Gain17/1
  Sum7/1 -> Sum2/1  "P/DC"
  PID Controller3/1 -> Delay2/1  "Id_ref_(nodelay)"
  [Delay] -> Delay2/2
  BW and PM Tester V/3(Visual Delay) -> delay V [s]/1
  BW and PM TesterP/DC/3(Visual Delay) -> delay P [s]/1
  Demux5/1 -> Terminator1/1  "vd"
  [V_sdq] -> Demux5/1
  Demux5/2 -> PID Controller5/1  "vq"
  Constant14/1 -> Sum8/2
  Sum8/1 -> Gain10/1, Integrator with Wrapped State (Discrete or Continuous)1/1  "w"
  PID Controller5/1 -> Sum8/1
  Integrator with Wrapped State (Discrete or Continuous)1/1 -> [rho]  "p"
  Mux/1 -> dq0 to abc/1  "v_dq0_ref"
  Gain10/1 -> [omega]
  [V_sdq] -> Demux6/1
  Demux6/1 -> PLL/1  "Vd_poc"
  Demux6/2 -> PLL/2  "Vq_poc"
  [omega] -> PLL/3  "Frequency"
  [rho] -> PLL/4  "Angle"
  Constant13/1 -> BW PLL/1
  Constant15/1 -> Phase Margin PLL/1
  Constant17/1 -> Ki PLL/1
  Constant16/1 -> Kp PLL/1
  [I_Ldq] -> Current source calculation and DC Voltage measurement/4(In3)
  Current source calculation and DC Voltage measurement/1(Out2) -> Controlled Current Source/1
  Current source calculation and DC Voltage measurement/2(Out1) -> Controlled Current Source1/1
  Current source calculation and DC Voltage measurement/3(Output) -> Gain11/1
  Memory4/1 -> [V_dc_mes]
  [V_rdq] -> Current source calculation and DC Voltage measurement/3(Input)
  [V_dc_mes] -> Current source calculation and DC Voltage measurement/2(In2)
  Voltage Measurement/1 -> Memory4/1
  P_ref/1 -> [P_ref], Sum7/2  "P_ref"
  [P_mes] -> Gain13/1  "P_mes"
  Sum9/1 -> Sum2/3, [Vdc_ref]  "Vdc_ref"
  [V_dc_pu] -> Sum7/3
  Gain11/1 -> [V_dc_pu]
  [Vdc_mes_pu] -> DC Voltage/1  "Measured Vdc"
  [Vdc_analyt] -> DC Voltage/2  "Analytical Vdc"
  Constant18/1 -> Phase Margin DC/1
  Constant19/1 -> BW Outer DC/1
  Constant21/1 -> Ki Outer (DC)/1
  Constant20/1 -> Kp Outer (DC)/1
  Power_Input/1 -> [Pm_ref], Current source calculation and DC Voltage measurement/1(In1)
  Vdc_ref/1 -> Sum9/2  "Vdc_ref"
  Gain16/1 -> Sum7/1
  Gain17/1 -> Sum9/1
  [Vdc_ref] -> Outer DC TF/1(In1)
  [Pm_ref] -> Outer DC TF/2(In2)
  Outer DC TF/1(Out1) -> [Vdc_analyt]
  Gain13/1 -> Sum2/2
  [V_dc_mes] -> Gain12/1
  Gain12/1 -> [Vdc_mes_pu]
  connections:
  Three-Phase Series RLC Branch/LConn1 -- Three-Phase V-I Measurement1/RConn1
  Three-Phase Series RLC Branch/LConn2 -- Three-Phase V-I Measurement1/RConn2
  Three-Phase Series RLC Branch/LConn3 -- Three-Phase V-I Measurement1/RConn3
  Three-Phase V-I Measurement2/LConn1 -- Three-Phase Series RLC Branch/RConn1 -- Three-Phase Series RLC Branch1/LConn1
  Three-Phase V-I Measurement2/LConn2 -- Three-Phase Series RLC Branch/RConn2 -- Three-Phase Series RLC Branch1/LConn2
  Three-Phase Series RLC Branch/RConn3 -- Three-Phase V-I Measurement2/LConn3 -- Three-Phase Series RLC Branch1/LConn3
  Ground/LConn1 -- Three-Phase Series RLC Branch1/RConn3 -- Three-Phase Series RLC Branch1/RConn1 -- Three-Phase Series RLC Branch1/RConn2
  Controlled Voltage Source/RConn1 -- Three-Phase V-I Measurement1/LConn1
  Controlled Voltage Source1/RConn1 -- Three-Phase V-I Measurement1/LConn2
  Controlled Voltage Source2/RConn1 -- Three-Phase V-I Measurement1/LConn3
  Controlled Voltage Source2/LConn1 -- Controlled Voltage Source1/LConn1 -- Controlled Voltage Source/LConn1
  Three-Phase V-I Measurement2/RConn1 -- Three-Phase Source/RConn1
  Three-Phase V-I Measurement2/RConn2 -- Three-Phase Source/RConn2
  Three-Phase V-I Measurement2/RConn3 -- Three-Phase Source/RConn3
  Voltage Measurement/LConn2 -- Controlled Current Source/LConn1 -- Parallel RLC Branch/RConn1 -- Controlled Current Source1/RConn1
  Parallel RLC Branch/LConn1 -- Controlled Current Source1/LConn1 -- Voltage Measurement/LConn1 -- Controlled Current Source/RConn1

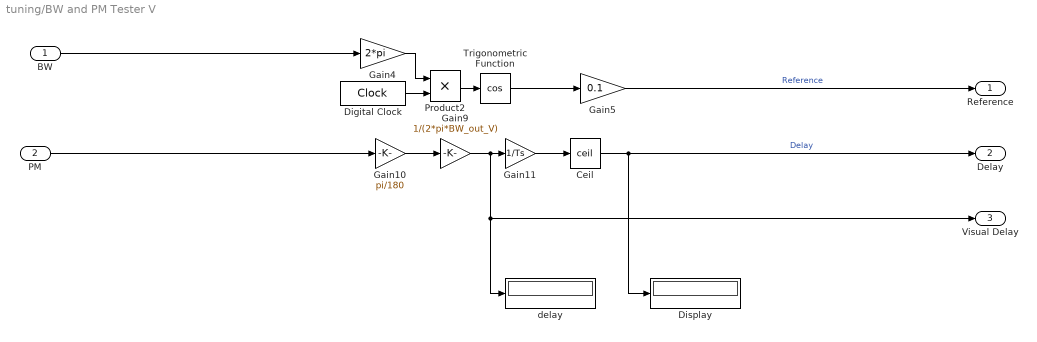
== system tuning/BW and PM Tester V ==
  BW : Inport
  PM : Inport  Port=2
  Ceil : Rounding  Operator=ceil
  Digital Clock : DigitalClock  SampleTime=Ts
  Display : Display
  Gain10 : Gain  Gain=pi/180
  Gain11 : Gain  Gain=1/Ts
  Gain4 : Gain  Gain=2*pi
  Gain5 : Gain  Gain=0.1
  Gain9 : Gain  Gain=1/(2*pi*BW_out_V)
  Product2 : Product
  Trigonometric Function : Trigonometry  Operator=cos
  delay : Display
  Reference : Outport
  Delay : Outport  Port=2
  Visual Delay : Outport  Port=3
  wires:
  Digital Clock/1 -> Product2/2
  Gain10/1 -> Gain9/1
  Gain11/1 -> Ceil/1
  Trigonometric Function/1 -> Gain5/1
  Gain9/1 -> delay/1, Visual Delay/1, Gain11/1
  Product2/1 -> Trigonometric Function/1
  Ceil/1 -> Delay/1, Display/1  "Delay"
  Gain4/1 -> Product2/1
  PM/1 -> Gain10/1
  Gain5/1 -> Reference/1  "Reference"
  BW/1 -> Gain4/1

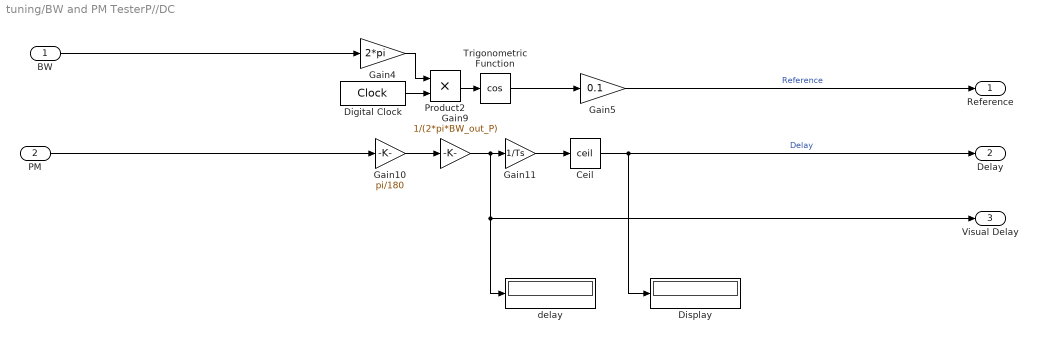
== system tuning/BW and PM TesterP//DC ==
  BW : Inport
  PM : Inport  Port=2
  Ceil : Rounding  Operator=ceil
  Digital Clock : DigitalClock  SampleTime=Ts
  Display : Display
  Gain10 : Gain  Gain=pi/180
  Gain11 : Gain  Gain=1/Ts
  Gain4 : Gain  Gain=2*pi
  Gain5 : Gain  Gain=0.1
  Gain9 : Gain  Gain=1/(2*pi*BW_out_P)
  Product2 : Product
  Trigonometric Function : Trigonometry  Operator=cos
  delay : Display
  Reference : Outport
  Delay : Outport  Port=2
  Visual Delay : Outport  Port=3
  wires:
  Digital Clock/1 -> Product2/2
  Gain10/1 -> Gain9/1
  Gain11/1 -> Ceil/1
  Trigonometric Function/1 -> Gain5/1
  Gain9/1 -> Visual Delay/1, delay/1, Gain11/1
  Product2/1 -> Trigonometric Function/1
  Ceil/1 -> Delay/1, Display/1  "Delay"
  Gain4/1 -> Product2/1
  PM/1 -> Gain10/1
  Gain5/1 -> Reference/1  "Reference"
  BW/1 -> Gain4/1

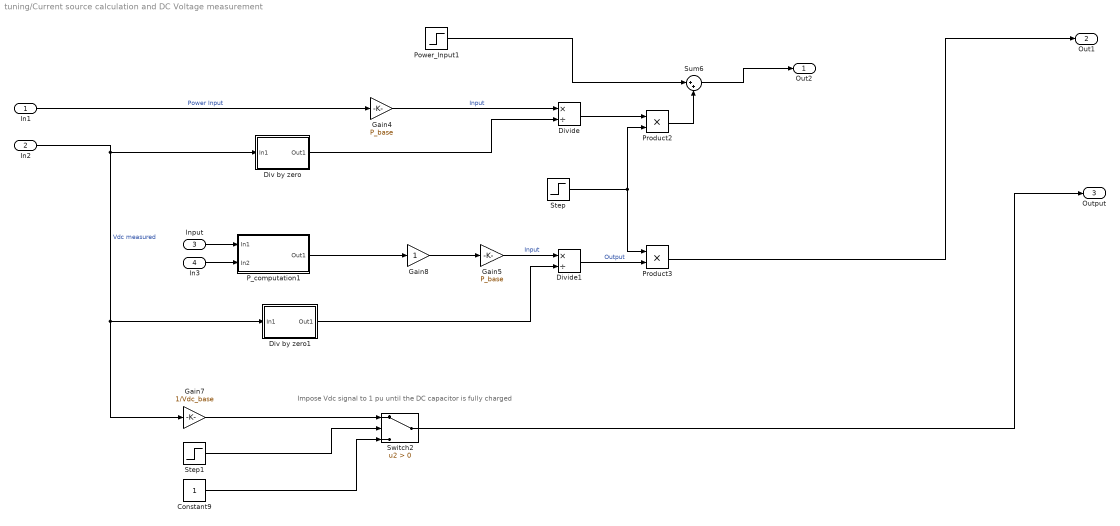
== system tuning/Current source calculation and DC Voltage measurement ==
  note: Impose Vdc signal to 1 pu until the DC capacitor is fully charged
  In1 : Inport
  In2 : Inport  Port=2
  Input : Inport  Port=3
  In3 : Inport  Port=4
  Constant9 : Constant
  Div by zero : Subsystem
  Div by zero1 : Subsystem
  Divide : Product  Inputs=*/
  Divide1 : Product  Inputs=*/
  Gain4 : Gain  Gain=P_base
  Gain5 : Gain  Gain=P_base
  Gain7 : Gain  Gain=1/Vdc_base
  Gain8 : Gain
  P_computation1 : Subsystem
  Power_Input1 : Step  Time=t_charge  Before=I_charge  After=0  SampleTime=0
  Product2 : Product
  Product3 : Product
  Step : Step  Time=t_charge + 0.1  SampleTime=0
  Step1 : Step  Time=t_charge + 0.1  SampleTime=0
  Sum6 : Sum  Inputs=|++
  Switch2 : Switch  Criteria=u2 > Threshold  SaturateOnIntegerOverflow=off  InputSameDT=off
  Out2 : Outport
  Out1 : Outport  Port=2
  Output : Outport  Port=3
  wires:
  In1/1 -> Gain4/1  "Power Input"
  Product3/1 -> Out1/1
  Step/1 -> Product3/1, Product2/2
  Divide/1 -> Product2/1
  Gain8/1 -> Gain5/1
  Divide1/1 -> Product3/2  "Output"
  Product2/1 -> Sum6/2
  Gain5/1 -> Divide1/1  "Input"
  Power_Input1/1 -> Sum6/1
  P_computation1/1(Out1) -> Gain8/1
  Gain4/1 -> Divide/1  "Input"
  Sum6/1 -> Out2/1
  Input/1 -> P_computation1/1(In1)
  In3/1 -> P_computation1/2(In2)
  Step1/1 -> Switch2/2
  Switch2/1 -> Output/1
  Gain7/1 -> Switch2/1
  In2/1 -> Gain7/1, Div by zero1/1(In1), Div by zero/1(In1)  "Vdc measured"
  Constant9/1 -> Switch2/3
  Div by zero/1(Out1) -> Divide/2
  Div by zero1/1(Out1) -> Divide1/2

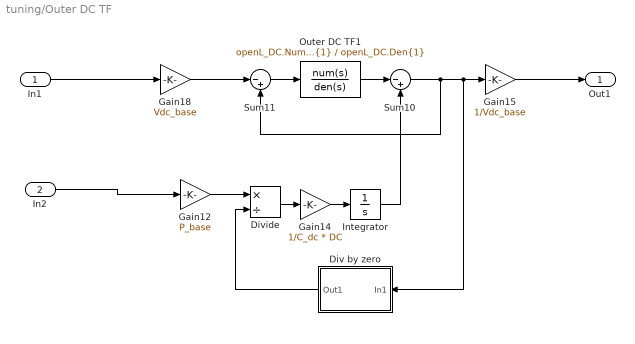
== system tuning/Outer DC TF ==
  In1 : Inport
  In2 : Inport  Port=2
  Div by zero : Subsystem
  Divide : Product  Inputs=*/
  Gain12 : Gain  Gain=P_base
  Gain14 : Gain  Gain=1/C_dc * DC
  Gain15 : Gain  Gain=1/Vdc_base
  Gain18 : Gain  Gain=Vdc_base
  Integrator : Integrator
  Outer DC TF1 : TransferFcn  Numerator=openL_DC.Num{1}  Denominator=openL_DC.Den{1}
  Sum10 : Sum  Inputs=|-+
  Sum11 : Sum  Inputs=|-+
  Out1 : Outport
  wires:
  Div by zero/1(Out1) -> Divide/2
  Sum10/1 -> Div by zero/1(In1), Gain15/1, Sum11/2
  Divide/1 -> Gain14/1
  In1/1 -> Gain18/1
  Outer DC TF1/1 -> Sum10/1
  Gain15/1 -> Out1/1
  Integrator/1 -> Sum10/2
  Gain14/1 -> Integrator/1
  Gain12/1 -> Divide/1
  Sum11/1 -> Outer DC TF1/1
  Gain18/1 -> Sum11/1
  In2/1 -> Gain12/1

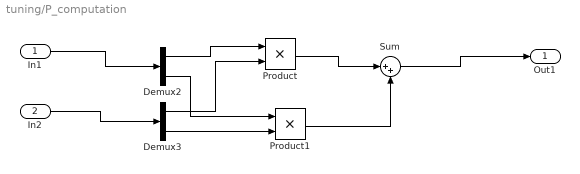
== system tuning/P_computation ==
  In1 : Inport
  In2 : Inport  Port=2
  Demux2 : Demux  Outputs=2
  Demux3 : Demux  Outputs=2
  Product : Product
  Product1 : Product
  Sum : Sum  Inputs=|++
  Out1 : Outport
  wires:
  In1/1 -> Demux2/1
  In2/1 -> Demux3/1
  Demux2/1 -> Product/1
  Demux3/1 -> Product/2
  Demux2/2 -> Product1/1
  Demux3/2 -> Product1/2
  Product/1 -> Sum/1
  Product1/1 -> Sum/2
  Sum/1 -> Out1/1

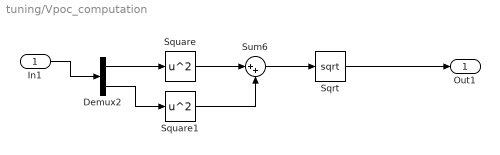
== system tuning/Vpoc_computation ==
  In1 : Inport
  Demux2 : Demux  Outputs=2
  Sqrt : Sqrt
  Square : Math  Operator=square
  Square1 : Math  Operator=square
  Sum6 : Sum  Inputs=|++
  Out1 : Outport
  wires:
  Sqrt/1 -> Out1/1
  Sum6/1 -> Sqrt/1
  Demux2/1 -> Square/1
  Square1/1 -> Sum6/2
  In1/1 -> Demux2/1
  Square/1 -> Sum6/1
  Demux2/2 -> Square1/1

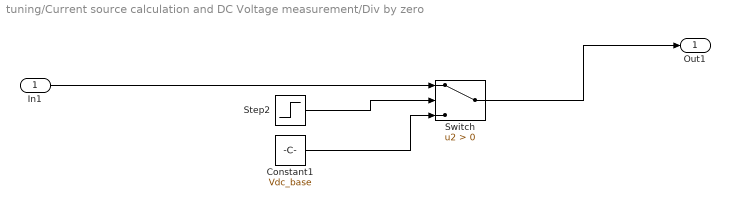
== system tuning/Current source calculation and DC Voltage measurement/Div by zero ==
  In1 : Inport
  Constant1 : Constant  Value=Vdc_base
  Step2 : Step  Time=0.1  SampleTime=0
  Switch : Switch  Criteria=u2 > Threshold  SaturateOnIntegerOverflow=off  InputSameDT=off
  Out1 : Outport
  wires:
  Switch/1 -> Out1/1
  Constant1/1 -> Switch/3
  In1/1 -> Switch/1
  Step2/1 -> Switch/2

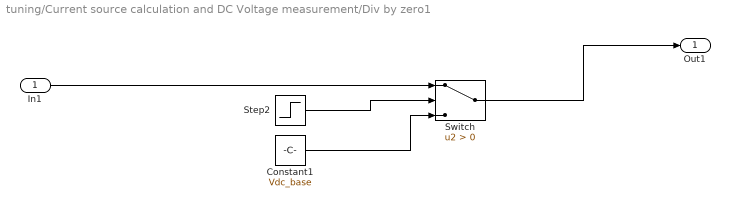
== system tuning/Current source calculation and DC Voltage measurement/Div by zero1 ==
  In1 : Inport
  Constant1 : Constant  Value=Vdc_base
  Step2 : Step  Time=0.1  SampleTime=0
  Switch : Switch  Criteria=u2 > Threshold  SaturateOnIntegerOverflow=off  InputSameDT=off
  Out1 : Outport
  wires:
  Step2/1 -> Switch/2
  In1/1 -> Switch/1
  Constant1/1 -> Switch/3
  Switch/1 -> Out1/1

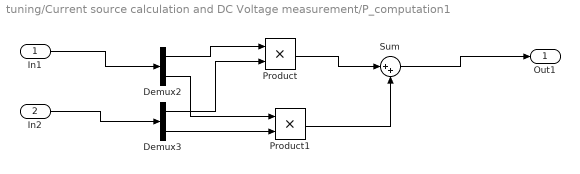
== system tuning/Current source calculation and DC Voltage measurement/P_computation1 ==
  In1 : Inport
  In2 : Inport  Port=2
  Demux2 : Demux  Outputs=2
  Demux3 : Demux  Outputs=2
  Product : Product
  Product1 : Product
  Sum : Sum  Inputs=|++
  Out1 : Outport
  wires:
  In1/1 -> Demux2/1
  In2/1 -> Demux3/1
  Demux2/1 -> Product/1
  Demux3/1 -> Product/2
  Demux2/2 -> Product1/1
  Demux3/2 -> Product1/2
  Product/1 -> Sum/1
  Product1/1 -> Sum/2
  Sum/1 -> Out1/1

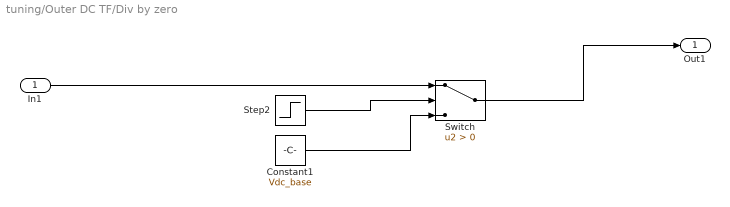
== system tuning/Outer DC TF/Div by zero ==
  In1 : Inport
  Constant1 : Constant  Value=Vdc_base
  Step2 : Step  Time=0.1  After=1*DC  SampleTime=0
  Switch : Switch  Criteria=u2 > Threshold  SaturateOnIntegerOverflow=off  InputSameDT=off
  Out1 : Outport
  wires:
  Switch/1 -> Out1/1
  Constant1/1 -> Switch/3
  In1/1 -> Switch/1
  Step2/1 -> Switch/2
